simulink library "HeatPump"  (R2018b)
settings: Solver=ode45  StartTime=0.0  StopTime=10.0  RelTol=1e-3  EnableMultiTasking=on
undefined symbols (not defined in the file): path_carnot, THBout_cold, THBout_hot
libraries: carnot x3
settings Model: Creator=lena.frank  LastModifiedBy=drhf
settings DataIOCC: LimitDataPoints=on  SaveFormat=Array  SignalLoggingSaveFormat=ModelDataLogs
settings OptimizationCC: ExpressionDepthLimit=2147483647  LifeSpan=inf
settings DebuggingCC: UnderspecifiedInitializationDetection=Classic  MergeDetectMultiDrivingBlocksExec=none  SolverPrmCheckMsg=warning  FcnCallInpInsideContextMsg=warning  StateNameClashWarn=warning  SFUnexpectedBacktrackingDiag=warning  SFNoUnconditionalDefaultTransitionDiag=warning  SFExecutionAtInitializationDiag=none
settings HardwareCC: ProdBitPerPointer=32  ProdBitPerSizeT=32  ProdBitPerPtrDiffT=32  ProdLargestAtomicFloat=None  ProdIntDivRoundTo=Undefined  ProdEndianess=Unspecified  ProdWordSize=32  ProdHWDeviceType=32-bit Generic
settings ModelReferenceCC: PropagateSignalLabelsOutOfModel=off
settings SFSimCC: SimUseLocalCustomCode=off
settings RTWCC: RTWUseLocalCustomCode=off
settings CodeAppCC: StateflowObjectComments=on
settings GRTTargetCC: TargetLangStandard=C89/C90 (ANSI)  GeneratePreprocessorConditionals=Disable all  CombineOutputUpdateFcns=off  GRTInterface=on
settings ConfigComp: CovMetricSettings=dw  CovHtmlReporting=on  CovSaveCumulativeToWorkspaceVar=on  CovSaveSingleToWorkspaceVar=on  CovExternalEMLEnable=off

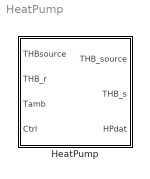
== system HeatPump ==
  HeatPump : Subsystem  mask(Heat Pump CONF){PathName=fullfile(path_carnot('libsl'), 'Source','Heat_Pump','HeatPump','parameter_set'), FileName='<user defined>', userPath=off, userParam=off, K=[300 -60 12250 -6.666666 60 -5.1315833e-05 306.66666 -115 12225], caph=32000, capc=32000, UA=6, relQdotMin=1, linc=10, quac=100, linh=10, quah=100}
      mask prompts: PathName "Path"; FileName "Parameter set"; userPath "Edit path and name of parameter set"; userParam "User defined parameters"; K "Parameters K (see also HP_param.m)"; caph "thermal capacity hot loop [J/K]"; capc "thermal capacity cold loop [J/K]"; UA "heat loss coefficient [W/K]"; relQdotMin "Minimum control signal for "on" (0...1)"; linc "cold side: linear pressure drop Pa/(kg/s)"; quac "cold side: quadratic pressure drop Pa/(kg/s)²"; linh "hot side : linear pressure drop Pa/(kg/s)"; quah "hot side: quadratic pressure drop Pa/(kg/s)²"
      mask help:
      | Configurated heat pump model, variables are defined in a mat-file (for example in "DefaultHeatPump.mat"). The linearized heat pump model uses measured data (e.g. EN 14511).
      | This block uses predefined parameter sets.
      | -   heating_power = K1 * Tprimary + K2 * Tsecondary + K3
      | -   electric_power = K4 * Tprimary + K5 * Tsecondary + K6
      | -   absorbing_power = K7 * Tprimary + K8 * Tsecondary + K9
      mask init:
      | % callback to set parameters of model
      | [ok, param] = CarnotCallbacks_HeatPump('SetParameters',gcbh,PathName,FileName);
      mask Help: web(fullfile(path_carnot('help'),'heatpump.html'),'-helpbrowser')
      mask Callback userPath: [ok, param] = CarnotCallbacks_HeatPump('UserEdit',gcbh);
      mask Callback userParam: [ok, param] = CarnotCallbacks_HeatPump('UserEdit',gcbh);
      mask TypeOptions K: HeatPump_basic/K
      mask TypeOptions caph: HeatPump_basic/caph
      mask TypeOptions capc: HeatPump_basic/capc
      mask TypeOptions UA: HeatPump_basic/UA
      mask TypeOptions relQdotMin: Switch/Threshold
      mask TypeOptions linc: Pressure_Drop_Cold/lin
      mask TypeOptions quac: Pressure_Drop_Cold/qua
      mask TypeOptions linh: Pressure_Drop_Hot/lin
      mask TypeOptions quah: Pressure_Drop_Hot/qua
      mask DialogControl Control1 Prompt: Carnot public data
      mask DialogControl Control1 Callback: [ok, file] = CarnotCallbacks_HeatPump('GetFilename',gcbh,'public');
      mask DialogControl Control3 Prompt: Carnot internal data
      mask DialogControl Control3 Callback: [ok, file] = CarnotCallbacks_HeatPump('GetFilename',gcbh,'internal');
      mask DialogControl Control4 Prompt: Selected path
      mask DialogControl Control4 Callback: [ok, file] = CarnotCallbacks_HeatPump('GetFilename',gcbh,'selected');
      mask DialogControl Container6 Prompt: HP Characteristic
      mask DialogControl Container7 Prompt: Hydraulic
      mask DialogControl Control5 Prompt: Save in Carnot internal data
      mask DialogControl Control5 Callback: [ok, param] = CarnotCallbacks_HeatPump('SaveFilename',gcbh,'internal','HP');
      mask DialogControl Control6 Prompt: Save in selected path
      mask DialogControl Control6 Callback: [ok, param] = CarnotCallbacks_HeatPump('SaveFilename',gcbh,'selected','HP');
      mask Display:
      | % user defined picture file
      | picfile = fullfile(path_carnot('intlibsl'), ...
      |     'Source','Heat_Pump','HeatPump','parameter_set', ...
      |     'HeatPump_CONF.jpg');
      | 
      | pic = false;
      | 
      | % show internal picture if defined
      | if ~BlockIsInCarnotLibrary    % if not located in library any more
      |     if exist(picfile)
      |         image(imread(picfile), [0.1, 0, 0.8, 1])
      |         set_param(gcb, 'BackgroundColor', 'White')
      |         pic = true;
      |     end
      | end
      | 
      | if ~pic   % show public picture
      |     set_param(gcb, 'BackgroundColor', 'Red')
      |     plot([10,20,40,60,80,90,90,80,60,40,20,10,10]/100, ...
      |         [60,80,90,90,80,60,40,20,10,10,20,40,60]/100,[40,20]/100,...
      |         [90,20]/100,[60,80]/100,[90,20]/100,[50,50]/100, ...
      |         [30,50]/100,[60,40]/100,[40,40]/100,...
      |         [57,43]/100,[33,46]/100,[44,57]/100,[34,46]/100)
      | end

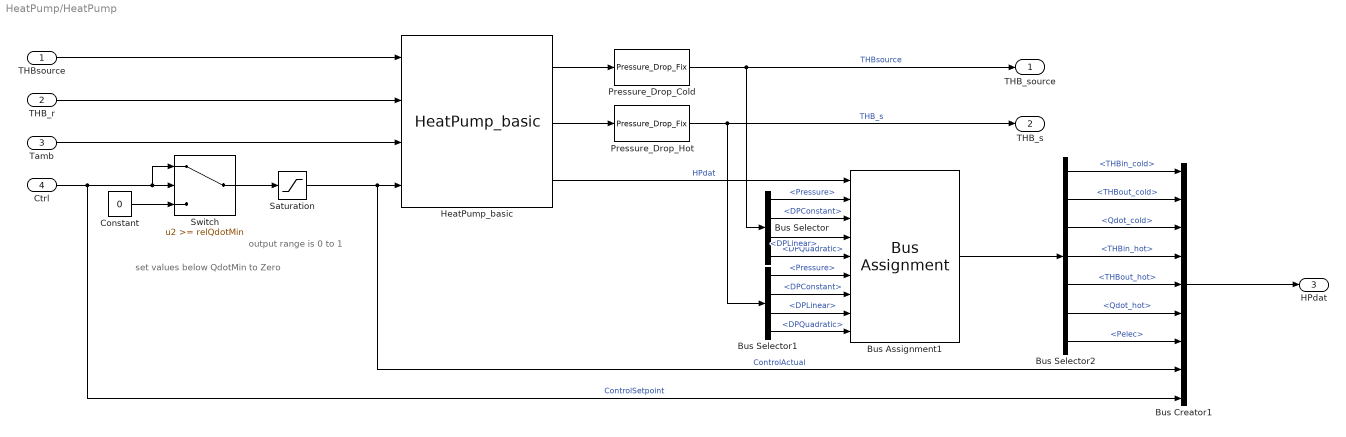
== system HeatPump/HeatPump ==
  note: set values below QdotMin to Zero
  note: output range is 0 to 1
  THBsource : Inport
  THB_r : Inport  Port=2
  Tamb : Inport  Port=3
  Ctrl : Inport  Port=4
  Bus Assignment1 : BusAssignment  AssignedSignals=THBout_cold.Pressure,THBout_cold.DPConstant,THBout_cold.DPLinear,THBout_cold.DPQuadratic,THBout_hot.Pressure,THBout_hot.DPConstant,THBout_hot.DPLinear,THBout_hot.DPQuadratic
  Bus Creator1 : BusCreator  Inputs=9
  Bus Selector : BusSelector  OutputSignals=Pressure,DPConstant,DPLinear,DPQuadratic
  Bus Selector1 : BusSelector  OutputSignals=Pressure,DPConstant,DPLinear,DPQuadratic
  Bus Selector2 : BusSelector  OutputSignals=THBin_cold,THBout_cold,Qdot_cold,THBin_hot,THBout_hot,Qdot_hot,Pelec
  Constant : Constant  Value=0
  HeatPump_basic : carnot/Basic/Thermal_Models/HeatPump_basic  K=K  caph=caph  capc=capc  UA=UA
      settings: SourceProductName=Carnot
  Pressure_Drop_Cold : carnot/Basic/Pressure_Drop/Pressure_Drop_Fix  con=0  lin=linc  qua=quac
      settings: SourceProductName=Carnot
  Pressure_Drop_Hot : carnot/Basic/Pressure_Drop/Pressure_Drop_Fix  con=0  lin=linh  qua=quah
      settings: SourceProductName=Carnot
  Saturation : Saturate  UpperLimit=1  LowerLimit=0
  Switch : Switch  Threshold=relQdotMin
  THB_source : Outport
  THB_s : Outport  Port=2
  HPdat : Outport  Port=3
  wires:
  Bus Selector1/4 -> Bus Assignment1/9  "<DPQuadratic>"
  Bus Selector1/3 -> Bus Assignment1/8  "<DPLinear>"
  Bus Selector1/2 -> Bus Assignment1/7  "<DPConstant>"
  Bus Selector1/1 -> Bus Assignment1/6  "<Pressure>"
  Bus Selector/4 -> Bus Assignment1/5  "<DPQuadratic>"
  Bus Selector/3 -> Bus Assignment1/4  "<DPLinear>"
  Bus Selector/2 -> Bus Assignment1/3  "<DPConstant>"
  Bus Selector/1 -> Bus Assignment1/2  "<Pressure>"
  HeatPump_basic/3 -> Bus Assignment1/1  "HPdat"
  Pressure_Drop_Cold/1 -> Bus Selector/1, THB_source/1  "THBsource"
  HeatPump_basic/1 -> Pressure_Drop_Cold/1
  Tamb/1 -> HeatPump_basic/3
  THB_r/1 -> HeatPump_basic/2
  THBsource/1 -> HeatPump_basic/1
  HeatPump_basic/2 -> Pressure_Drop_Hot/1
  Pressure_Drop_Hot/1 -> Bus Selector1/1, THB_s/1  "THB_s"
  Constant/1 -> Switch/3
  Switch/1 -> Saturation/1
  Bus Selector2/7 -> Bus Creator1/7  "<Pelec>"
  Bus Selector2/4 -> Bus Creator1/4  "<THBin_hot>"
  Bus Creator1/1 -> HPdat/1
  Bus Selector2/5 -> Bus Creator1/5  "<THBout_hot>"
  Bus Assignment1/1 -> Bus Selector2/1
  Bus Selector2/3 -> Bus Creator1/3  "<Qdot_cold>"
  Bus Selector2/6 -> Bus Creator1/6  "<Qdot_hot>"
  Ctrl/1 -> Bus Creator1/9, Switch/1, Switch/2  "ControlSetpoint"
  Bus Selector2/2 -> Bus Creator1/2  "<THBout_cold>"
  Saturation/1 -> Bus Creator1/8, HeatPump_basic/4  "ControlActual"
  Bus Selector2/1 -> Bus Creator1/1  "<THBin_cold>"
